simulink model "fluid_system"  (R2023a)
settings: Solver=FixedStepAuto  StartTime=0.0  StopTime=1000  FixedStep=0.1  RelTol=1e-3
settings Model: Creator=Lucca  LastModifiedBy=Lucca
settings SolverCC: ZeroCrossAlgorithm=Adaptive
settings DebuggingCC: IgnoredZcDiagnostic=none

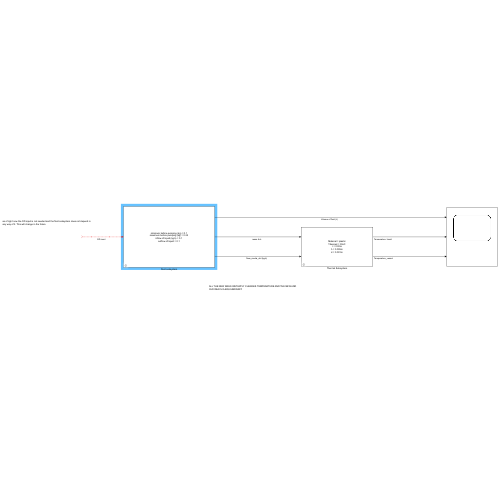
[thumbnail: Simulink's stored preview of the top-level diagram]
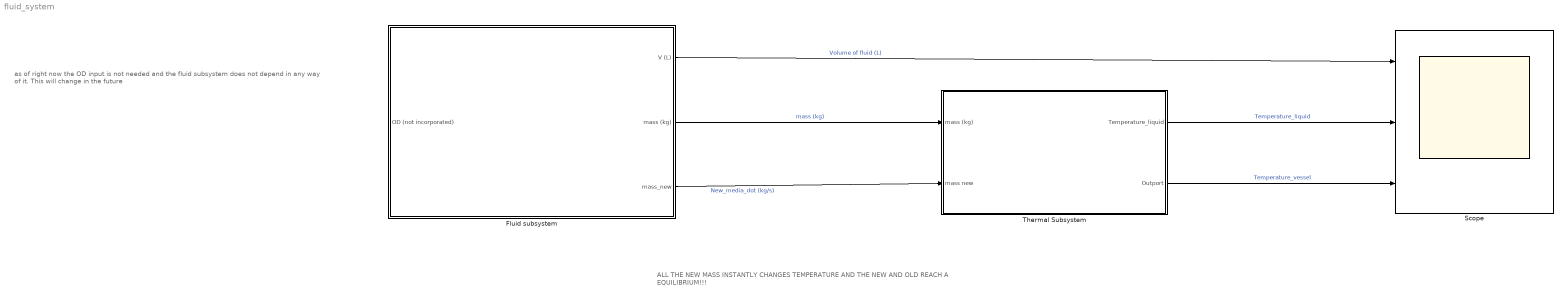
== system fluid_system ==
  note: as of right now the OD input is not needed and the fluid subsystem does not depend in any way of it. This will change in the future
  note: ALL THE NEW MASS INSTANTLY CHANGES TEMPERATURE AND THE NEW AND OLD REACH A EQUILIBRIUM!!!
  Fluid subsystem : Subsystem  mask{min=0.1, max=0.25, in_flow=0.02, out_flow=0.02, density=1}
      mask prompts: min "minimum mass of liquid (kg)"; max "maximum mass of liquid (kg)"; in_flow "flow of liquid in (kg/s)"; out_flow "flow of liquid out (kg/s)"; density "density of liquid (kg/dm^3)"
      mask init:
      | str0 = "minimum before pumping (kg) = " + min;
      | str1 = "maximum before pumping (kg) = " + max;
      | str2 = "inflow of liquid (kg/s) = " + min;
      | str3 = "outflow of liquid = " + min;
      | 
      | label  = [str0;str1;str2;str3];
      mask Display: disp(label);
  Scope : Scope  NumInputPorts=3
  Thermal Subsystem : Subsystem  mask{material=plastic, r=0.02, h=0.005, d=0.001, ml=0.25, cl=4180, Tenv=25, Tf=30, mv=2, Pheat=100}
      mask prompts: material "Material of the walls"; r "r - radius of vessel (m)"; h "h - height of vessel (m)"; d "d - width of the vessel (m)"; ml "ml - mass of liquid (kg)"; cl "cl - specific heat of liquid (J/kg*K)"; Tenv "Tenv -  Ambient temperature (Celsiums)"; Tf "Tf - Desired final temperature (Celsiums)"; mv "mv - mass of vessel (kg)"; Pheat "Pheat - power of heating element (W)"
      mask init:
      | str01 = "Material = " + material;
      | str0 = "Tdesired = " + Tf + "oC";
      | str1 = "r = " + r + "m";
      | str2 = "h = " + h + "m";
      | str3 = "d = " + d + "m";
      | label = [str01; str0; str1; str2; str3];
      | 
      | switch material
      |     case 'plastic'
      |         cv = 1670;
      |         k = 0.3;
      |     case 'aluminium'
      |         cv = 897;
      |         k = 237;
      |     case 'glass'
      |         cv = 840;
      |         k = 1;
      |     case 'new material (change in code)'
      |         cv = 1;
      |         k = 1;
      |         
      |         
      |         
      | end
      mask TypeOptions material: plastic | aluminium | glass | new material (change in code)
      mask Display: disp(label);
  wires:
  Fluid subsystem/1(V (L)) -> Scope/1  "Volume of fluid (L)"
  Fluid subsystem/2(mass (kg)) -> Thermal Subsystem/1(mass (kg))  "mass (kg)"
  ? -> Fluid subsystem/1(OD (not incorporated))  "OD input"
  Fluid subsystem/3(mass_new) -> Thermal Subsystem/2(mass new)  "New_media_dot (kg/s)"
  Thermal Subsystem/1(Temperature_liquid) -> Scope/2  "Temperature_liquid"
  Thermal Subsystem/2(Outport) -> Scope/3  "Temperature_vessel"

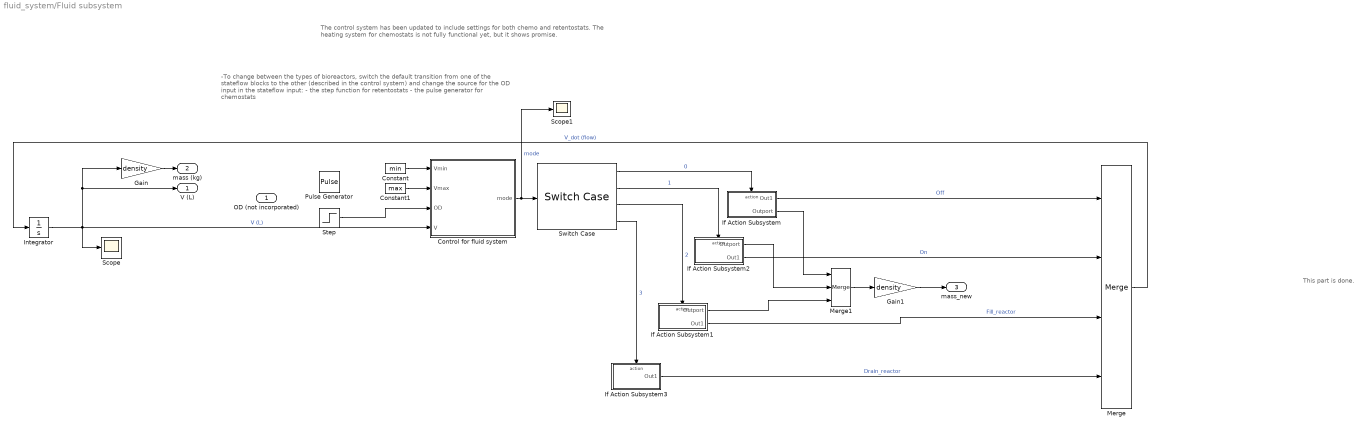
== system fluid_system/Fluid subsystem ==
  note: -To change between the types of bioreactors, switch the default transition from one of the stateflow blocks to the other (described in the control system) and change the source for the OD input in the stateflow input:
      |
      | - the step function for retentostats
      | - the pulse generator for chemostats
  note: The control system has been updated to include settings for both chemo and retentostats. The heating system for chemostats is not fully functional yet, but it shows promise.
  note: This part is done.
  OD (not incorporated) : Inport
  Constant : Constant  Value=min
  Constant1 : Constant  Value=max
  Control for fluid system : Stateflow chart  TreatAsAtomicUnit=on
  Gain : Gain  Gain=density
  Gain1 : Gain  Gain=density
  If Action Subsystem : Subsystem  TreatAsAtomicUnit=on
  If Action Subsystem1 : Subsystem  TreatAsAtomicUnit=on
  If Action Subsystem2 : Subsystem  TreatAsAtomicUnit=on
  If Action Subsystem3 : Subsystem  TreatAsAtomicUnit=on
  Integrator : Integrator  InitialCondition=0.1
  Merge : Merge  Inputs=4
  Merge1 : Merge  Inputs=3
  Pulse Generator : DiscretePulseGenerator  PulseType=Time based  Period=30  PulseWidth=10
  Scope : Scope
  Scope1 : Scope
  Step : Step  SampleTime=300
  Switch Case : SwitchCase  CaseConditions={0,1,2,3}  ShowDefaultCase=off
  V (L) : Outport
  mass (kg) : Outport  Port=2
  mass_new : Outport  Port=3
  wires:
  Switch Case/2 -> If Action Subsystem2/Action  "1"
  Switch Case/1 -> If Action Subsystem/Action  "0"
  Control for fluid system/1(mode) -> Scope1/1, Switch Case/1  "mode"
  If Action Subsystem/1(Out1) -> Merge/1  "Off"
  If Action Subsystem2/2(Out1) -> Merge/2  "On"
  If Action Subsystem1/2(Out1) -> Merge/3  "Fill_reactor"
  Integrator/1 -> Scope/1, Gain/1, V (L)/1, Control for fluid system/4(V)  "V (L)"
  Merge/1 -> Integrator/1  "V_dot (flow)"
  Constant/1 -> Control for fluid system/1(Vmin)
  Constant1/1 -> Control for fluid system/2(Vmax)
  Gain/1 -> mass (kg)/1
  Switch Case/3 -> If Action Subsystem1/Action  "2"
  Gain1/1 -> mass_new/1
  If Action Subsystem2/1(Outport) -> Merge1/2
  If Action Subsystem/2(Outport) -> Merge1/1
  Merge1/1 -> Gain1/1
  Switch Case/4 -> If Action Subsystem3/Action  "3"
  If Action Subsystem3/1(Out1) -> Merge/4  "Drain_reactor"
  If Action Subsystem1/1(Outport) -> Merge1/3
  Step/1 -> Control for fluid system/3(OD)

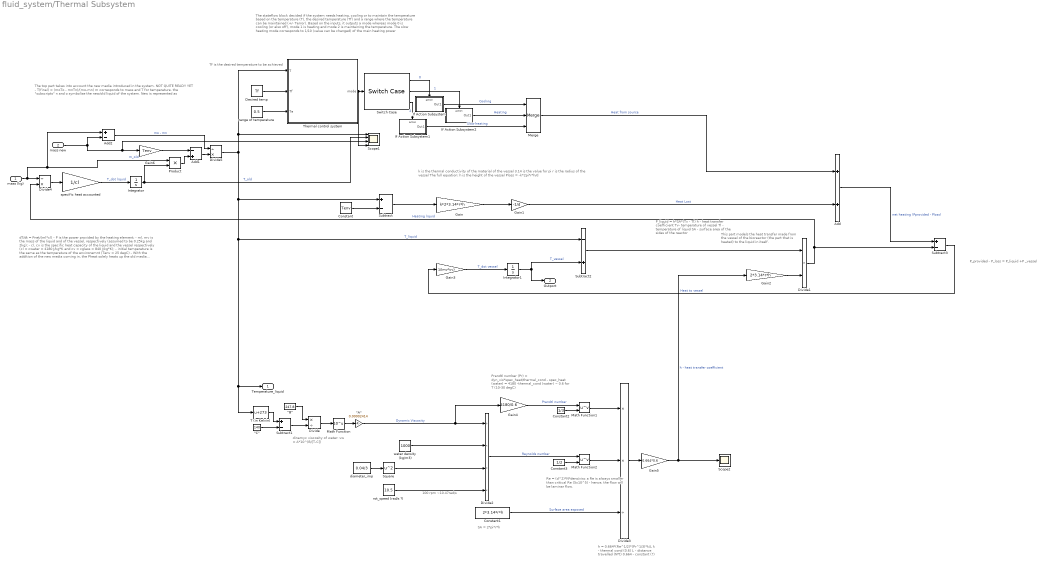
== system fluid_system/Thermal Subsystem ==
  note: The top part takes into account the new media introduced in the system. NOT QUITE READY YET
      |
      | - T(final) = (moTo - mnTn)/(mo-mn)
      |
      | m corresponds to mass and T for temperature. the "subscripts" n and o symbolise the new/old liquid of the system. New is represented as
  note: This part models the heat transfer made from the vessel of the bioreactor (the part that is heated) to the liquid in itself.
  note: P_liquid = h*SA*(Tv - Tl)
      |
      | h - heat transfer coefficient
      | Tv- temperature of vessel
      | Tl - temperature of liquid
      | SA - surface area of the sides of the reactor
  note: SA = 2*pi*r*h
  note: P_provided - P_loss = P_liquid +P _vessel
  note: dinamyc viscosity of water:
      | vw = A*10^(B/[T-C])
  note: The stateflow block decided if the system needs heating, cooling or to maintain the temperature based on the temperature (T), the desired temperature (Tf) and a range where the temperature can be maintained (+/- Terror).
      |
      | Based on the inputs, it outputs a mode whereas mode 0 is cooling (or also off), mode 1 is heating and mode 2 is maintaining the temperature.
      |
      | The slow heating mode corresponds to 1/10 (value can be changed) of the main heating power
  note: Tf is the desired temperature to be achieved
  note: dT/dt = Pnet/(ml*cl)
      |
      | - P is the power provided by the heating element;
      | - ml, mv is the mass of the liquid and of the vessel, respectively (assumed to be 0.25kg and 2kg);
      | - cl, cv is the specific heat capacity of the liquid and the vessel respectively (cl = cwater = 4180 J/kg*K and cv = cglass = 840 J/kg*K);
      | - initial temperature is the same as the temperature of the environemnt (Tenv = 25 degC)
      |
      | - With the addition of the new media coming in, the Pheat solely heats up the old media present in the vessel. The old media, alongside its temperature (that has already risen) will then be used to calculate the new averaged temperature with the new "colder" media that has been introduced.
      | - This function doesn't completely work when dealing with chemostats, however, it shows promise with retentostats.
  note: k is the thermal conductivity of the material of the vessel
      | 3.14 is the value for pi
      | r is the radius of the vessel The full equation:
      | h is the height of the vessel Ploss = -k*2pi*r*h/d
  note: Prandtl number (Pr) = dyn_vis*spec_heat/thermal_cond
      |
      | - spec_heat (water) = 4180
      | -thermal_cond (water) ~ 0.6 for T (10-30 degC)
  note: Re = (d^2)*N*dens/visc
      | a
      | Re is always smaller than critical Re (5x10^5)
      | - hence, the flow will be laminar flow.
  note: h = 0.664*(Re^1/2)*(Pr^1/3)*k/L
      | k - thermal cond (0.6)
      | L - distance travelled (N*t)
      | 0.664 - constant (?)
  note: 100 rpm ~10.47rad/s
  mass (kg) : Inport
  mass new : Inport  Port=2
  "\"A\"" : Gain  Gain=0.00002414
  "\"B\"" : Constant  Value=247.8
  "\"C\"" : Constant  Value=140
  Add : Sum
  Add1 : Sum  Inputs=-+
  Add2 : Sum  Inputs=+-
  Constant : Constant  Value=Tenv
  Constant1 : Constant  Value=2*3.14*r*h
  Constant2 : Constant  Value=1/3
  Constant3 : Constant  Value=1/2
  Desired temp : Constant  Value=Tf
  Divide : Product  Inputs=*/
  Divide1 : Product  Inputs=**
  Divide2 : Product  Inputs=/***
  Divide3 : Product  Inputs=**/
  Divide4 : Product  Inputs=/*
  Divide5 : Product  Inputs=/*
  Gain : Gain  Gain=k*2*3.14*r*h
  Gain1 : Gain  Gain=-1/d
  Gain2 : Gain  Gain=2*3.14*r*h
  Gain3 : Gain  Gain=1/(mv*cv)
  Gain4 : Gain  Gain=4180/0.6
  Gain5 : Gain  Gain=0.664*0.6
  Gain6 : Gain  Gain=Tenv
  If Action Subsystem : Subsystem  TreatAsAtomicUnit=on
  If Action Subsystem1 : Subsystem  TreatAsAtomicUnit=on
  If Action Subsystem2 : Subsystem  TreatAsAtomicUnit=on
  Integrator : Integrator  InitialCondition=Tenv
  Integrator1 : Integrator  InitialCondition=Tenv
  Math Function : Math  Operator=10^u
  Math Function1 : Math  Operator=pow
  Math Function2 : Math  Operator=pow
  Merge : Merge  Inputs=3
  Product : Product
  Scope1 : Scope  NumInputPorts=4
  Scope2 : Scope
  Square : Math  Operator=square
  Subtract : Sum  Inputs=+-
  Subtract1 : Sum  Inputs=+-
  Subtract2 : Sum  Inputs=-+
  Subtract3 : Sum  Inputs=+-
  Switch Case : SwitchCase  CaseConditions={0,1,2}  ShowDefaultCase=off
  T (in Kelvin) : Bias  Bias=273  SaturateOnIntegerOverflow=off
  Thermal control system : Stateflow chart  TreatAsAtomicUnit=on
  diameter_imp : Constant  Value=0.04/3
  range of temperature : Constant  Value=0.5
  rot_speed (rad/s ?) : Constant  Value=10.5
  specific heat accounted : Gain  Gain=1/cl
  "water density (kg/m3) " : Constant  Value=1000
  Temperature_liquid : Outport
  Outport : Outport  Port=2
  wires:
  Switch Case/3 -> If Action Subsystem1/Action  "2"
  Thermal control system/1(mode) -> Scope1/4, Switch Case/1
  Desired temp/1 -> Thermal control system/2(Tf)
  If Action Subsystem2/1(Out1) -> Merge/2  "Heating"
  specific heat accounted/1 -> Integrator/1  "T_dot liquid"
  Switch Case/2 -> If Action Subsystem2/Action  "1"
  If Action Subsystem/1(Out1) -> Merge/1  "Cooling"
  If Action Subsystem1/1(Out1) -> Merge/3  "Slow heating"
  Switch Case/1 -> If Action Subsystem/Action  "0"
  range of temperature/1 -> Thermal control system/3(Te)
  Merge/1 -> Add/1  "Heat from source"
  Constant/1 -> Subtract/2
  Subtract/1 -> Gain/1
  Gain/1 -> Gain1/1
  Gain1/1 -> Add/2  "Heat Lost"
  T (in Kelvin)/1 -> Subtract1/1
  "\"C\""/1 -> Subtract1/2
  Subtract1/1 -> Divide/2
  "\"B\""/1 -> Divide/1
  Divide/1 -> Math Function/1
  Math Function/1 -> "\"A\""/1
  Gain3/1 -> Integrator1/1  "T_dot vessel"
  Integrator1/1 -> Outport/1, Subtract2/2  "T_vessel"
  Subtract2/1 -> Divide1/1
  Gain2/1 -> Divide1/2
  Divide1/1 -> Subtract3/2, Divide4/2  "Heating liquid"
  Add/1 -> Subtract3/1  "net heating (Pprovided - Ploss)"
  Subtract3/1 -> Gain3/1  "Heat to vessel"
  Constant1/1 -> Divide3/3  "Surface area exposed"
  Math Function2/1 -> Divide3/2
  Constant3/1 -> Math Function2/2
  diameter_imp/1 -> Square/1
  Gain4/1 -> Math Function1/1  "Prandtl number"
  Math Function1/1 -> Divide3/1
  Divide2/1 -> Math Function2/1  "Reynolds number"
  Divide3/1 -> Gain5/1
  "water density (kg/m3) "/1 -> Divide2/2
  Gain5/1 -> Scope2/1, Gain2/1  "h - heat transfer coefficient"
  Square/1 -> Divide2/3
  rot_speed (rad/s ?)/1 -> Divide2/4
  Constant2/1 -> Math Function1/2
  "\"A\""/1 -> Divide2/1, Gain4/1  "Dynamic Viscosity"
  Divide4/1 -> specific heat accounted/1
  Gain6/1 -> Add1/1
  Product/1 -> Add1/2
  Add1/1 -> Divide5/2
  Add2/1 -> Divide5/1  "mo - mn"
  mass new/1 -> Scope1/3, Gain6/1, Add2/2
  Integrator/1 -> Scope1/2, Product/2  "T_old"
  mass (kg)/1 -> Add2/1, Product/1, Divide4/1  "m_old"
  Divide5/1 -> Temperature_liquid/1, T (in Kelvin)/1, Subtract2/1, Subtract/1, Scope1/1, Thermal control system/1(T)  "T_liquid"

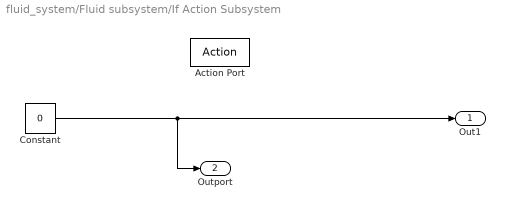
== system fluid_system/Fluid subsystem/If Action Subsystem ==
  Action Port : ActionPort  ActionPortLabel=case [ 0 ]:
  Constant : Constant  Value=0
  Out1 : Outport
  Outport : Outport  Port=2
  wires:
  Constant/1 -> Outport/1, Out1/1

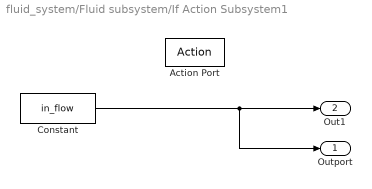
== system fluid_system/Fluid subsystem/If Action Subsystem1 ==
  Action Port : ActionPort  ActionPortLabel=case [ 2 ]:
  Constant : Constant  Value=in_flow
  Outport : Outport
  Out1 : Outport  Port=2
  wires:
  Constant/1 -> Outport/1, Out1/1

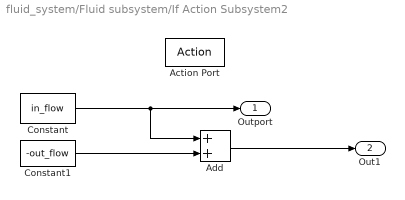
== system fluid_system/Fluid subsystem/If Action Subsystem2 ==
  Action Port : ActionPort  ActionPortLabel=case [ 1 ]:
  Add : Sum
  Constant : Constant  Value=in_flow
  Constant1 : Constant  Value=-out_flow
  Outport : Outport
  Out1 : Outport  Port=2
  wires:
  Constant/1 -> Outport/1, Add/1
  Constant1/1 -> Add/2
  Add/1 -> Out1/1

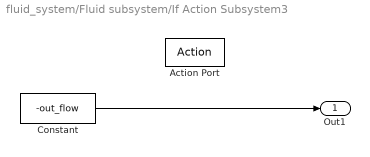
== system fluid_system/Fluid subsystem/If Action Subsystem3 ==
  Action Port : ActionPort  ActionPortLabel=case [ 3 ]:
  Constant : Constant  Value=-out_flow
  Out1 : Outport
  wires:
  Constant/1 -> Out1/1

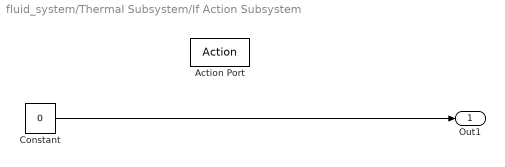
== system fluid_system/Thermal Subsystem/If Action Subsystem ==
  Action Port : ActionPort  ActionPortLabel=case [ 0 ]:
  Constant : Constant  Value=0
  Out1 : Outport
  wires:
  Constant/1 -> Out1/1

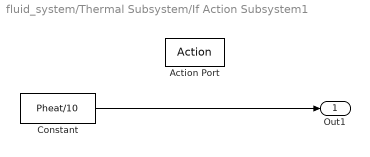
== system fluid_system/Thermal Subsystem/If Action Subsystem1 ==
  Action Port : ActionPort  ActionPortLabel=case [ 2 ]:
  Constant : Constant  Value=Pheat/10
  Out1 : Outport
  wires:
  Constant/1 -> Out1/1

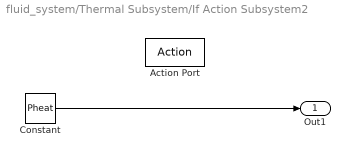
== system fluid_system/Thermal Subsystem/If Action Subsystem2 ==
  Action Port : ActionPort  ActionPortLabel=case [ 1 ]:
  Constant : Constant  Value=Pheat
  Out1 : Outport
  wires:
  Constant/1 -> Out1/1

== stateflow chart fluid_system/Thermal Subsystem/Thermal control system ==
  state Heating
    entry:
    mode = 1;
  state Cooling
    entry:
    mode = 0;
  state Slow_Heating
    entry:
    mode = 2;
  note: This part of the transition between cooling and slow heating can be observed to be changed (to save power, the slow heating part can be disabled after it reaches a certain temperature)
  (default) -> Cooling
  Cooling -> Heating [order 1] : [T < (Tf-Te) ]
  Heating -> Cooling [order 2] : [T > (Tf+Te)]
  Cooling -> Slow_Heating [order 2] : [T < Tf]
  Slow_Heating -> Cooling [order 2] : [T > Tf]
  Heating -> Slow_Heating [order 1] : [T > (Tf-Te)]
  Slow_Heating -> Heating [order 1] : [T < (Tf-Te)]
  data: T input; Tf input; mode output; Te input

== stateflow chart fluid_system/Fluid subsystem/Control for fluid system ==
  note: This part will work for retentostats (add the ball to off)
  note: This part will work for chemostats (add the ball to off_in)
  state Off
    entry:
    mode = 0;
  state On
    entry:
    mode = 1;
  note: This works for batch reactors! Not what we are doing
  state Off_in
    en:
    mode = 0;
  state Pump_in
    en:
    mode = 2;
  state Reactor_fill
    mode = 2;
  state Pump_out
    en:
    mode = 3;
  (default) -> Off
  Off -> On [order 1] : [OD == 1]
  On -> Off : [OD == 0]
  Off_in -> Pump_in [order 1] : [V <= Vmin]
  Off -> Reactor_fill [order 2] : [V <= Vmax]
  Reactor_fill -> Off : [V >= Vmax]
  Pump_in -> Off_in : [V >= Vmax]
  Off_in -> Pump_out [order 2] : [OD == 1]
  Pump_out -> Pump_in : [V <= Vmin]
  data: mode output =0; Vmin input; Vmax input; OD input; V input
